simulink model "E1"  (R2023a)
settings: Solver=VariableStepAuto  StartTime=0.0  StopTime=20  MaxStep=1e-4  RelTol=1e-3
settings Model: Creator=swara  LastModifiedBy=swara

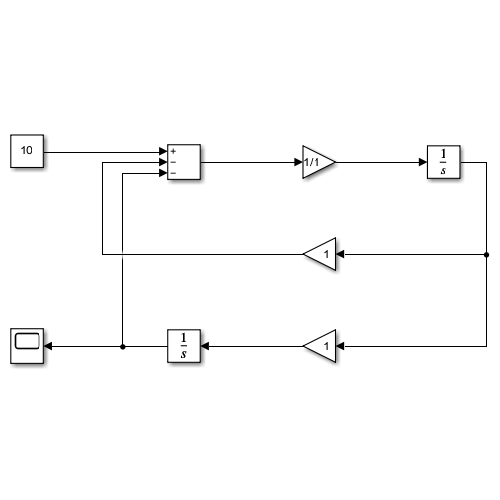
[thumbnail: Simulink's stored preview of the top-level diagram]
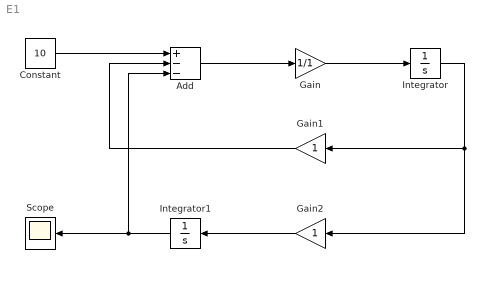
== system E1 ==
  Add : Sum  Inputs=+--
  Constant : Constant  Value=10
  Gain : Gain  Gain=1/1
  Gain1 : Gain
  Gain2 : Gain
  Integrator : Integrator
  Integrator1 : Integrator
  Scope : Scope
  wires:
  Constant/1 -> Add/1
  Add/1 -> Gain/1
  Gain/1 -> Integrator/1
  Gain1/1 -> Add/2
  Integrator/1 -> Gain1/1, Gain2/1
  Gain2/1 -> Integrator1/1
  Integrator1/1 -> Scope/1, Add/3
